simulink model "AssembledTEST1"  (R2016b)
settings: Solver=VariableStepAuto  StartTime=0.0  StopTime=60  RelTol=1e-9
values from neighbouring files (symbols this model uses):
  DOWN_0 = -xtrim(12)    [Comparison_NonLin.m]    (also in InitialiseJ31.m = 1830.0192; Trim.m)
  EAST_0 = xtrim(11)    [Comparison_NonLin.m]    (also in InitialiseJ31.m = 0; Trim.m)
  FLAP = 0    [InitialiseJ31.m]
  INERTIA = [IXX,IXY,IXZ;IXY,IYY,IYZ;IXZ,IYZ,IZZ]    [InitialiseJ31.m]
  NORTH_0 = xtrim(10)    [Comparison_NonLin.m]    (also in InitialiseJ31.m = 0; Trim.m)
  P_0 = xtrim(4)    [Comparison_NonLin.m]    (also in InitialiseJ31.m = 0; Trim.m)
  PHI_0 = xtrim(7)    [Comparison_NonLin.m]    (also in Trim.m)
  PSI_0 = xtrim(9)    [Comparison_NonLin.m]    (also in Trim.m)
  Q_0 = xtrim(5)    [Comparison_NonLin.m]    (also in InitialiseJ31.m = 0; Trim.m)
  R2D = 180/pi    (= 57.2957795131)    [InitialiseJ31.m]
  R_0 = xtrim(6)    [Comparison_NonLin.m]    (also in InitialiseJ31.m = 0; Trim.m)
  THETA_0 = xtrim(8)    [Comparison_NonLin.m]    (also in Trim.m)
  U_0 = xtrim(1)    [Comparison_NonLin.m]    (also in Trim.m)
  V_0 = xtrim(2)    [Comparison_NonLin.m]    (also in Trim.m)
  W_0 = xtrim(3)    [Comparison_NonLin.m]    (also in Trim.m)
undefined symbols (not defined in the file or in its folder): ail_data, Ap, Aw, b, beta0_data, c0, c_i, cdrag_data, CG, clean_wing_data, crt, CT_data, D, D0q_10, D0q_20, D0q_35, DCDi_data, DCM0b, Deh_f_on_data, Deh_on_data, df, Dqhq_data, e0, e_data10, e_data20, e_data35, elaw_0, elaw_1, elaw_2, flaps_lift_data, flaps_moment_data, flaps_tail_data, flaps_wing_data, fmc_data, fmf_data, fmn_data, fus_data, gamma_t, h_data10, h_data20, h_data35, it, iw, Iwn2, J_W, K1_data, k1f_data, k_data, L_r0_10f, L_r0_20f, L_r0_35f, l_t, ld_data, Lt, Lt_dash, Lv_b, Lv_h, Lv_n, mac, mach_ffr ... (+39)
libraries: aerolibasang x3, aerolibatmos2 x1
(part 5 of 5)

== matlab function AssembledTEST1/Subsystem/Lateral//Directional Aerodynamics/getYLN/Embedded MATLAB Function ==
  data: sigma input; Lv_b input; alpha input; Yv output; Yv_f input; Yv_v input; Y_rud input; Lv_di input; Lv_w_CL input; Np_w_CL input; Yp_w_CL input; a1_wb input; Lp_w input; CLw input; CLb input; Yv_wb input; Yv_n input; Yr_b input; Lv_n input; Lv_h input; Nv_wb input; Nv_n input; Nr_b input; J_W input; Yp output; Yr output; Y_zeta output; Lv output; Lp output; Lr output; L_zeta output; Nv output; Lr_0_f input; Lr_Lr0 input; Np output; Nr output; N_zeta output; b input; CD0w input; DelCDi_flap input; DelCD0_flap input
function [Yv,Yp,Yr,Y_zeta,Lv,Lp,Lr,L_zeta,Nv,Np,Nr,N_zeta] = Get_YLNderivs(sigma,Lv_b,alpha,Yv_f,Yv_v,Y_rud,Lv_di,Lv_w_CL,Np_w_CL,Yp_w_CL,a1_wb,Lp_w,CLw,CLb,Yv_wb,Yv_n,Yr_b,Lv_n,Lv_h,Nv_wb,Nv_n,Nr_b,J_W,Lr_0_f,Lr_Lr0,b,CD0w,DelCDi_flap,DelCD0_flap)

%CL_w,Dv_wing,D0_wing,p,q,r,Mach,V,alpha,beta,qbar,Aileron_L,Aileron_R,Rudder,Flap,wdot,xcg)

%   This function determines the side force, rolling momement and yawing
%   moment at the specified dynamic pressure.
%   Uses the methods given in ESDU 79006, 82010, 87008, 81013, 80033,
%   80034, 00025, 73006, A.06.01.03, 83006, 92029, 72021, 83026, 82017,
%   88029
%
%   Author: A Cooke Date:   1 Jun 05, modified 12 Jan 06, 16 Jun 06
%   Converted to embedded MatLab Function 31 Oct 07

% Yv_f  = sideforce derivative for fin 
Lv_f    =  (Yv_f/b) * (1.571 * cos(alpha) - 6.339 * sin(alpha));   % rolling moment derivative for fin
Nv_f    = -(Yv_f/b) * (6.339 * cos(alpha) + 1.571 * sin(alpha));   % yawing moment derivative for fin

% Yv_v  = sideforce derivative for ventral fin 
Lv_v    = -(Yv_v/b) * (0.524 * cos(alpha) + 6.335 * sin(alpha));   % rolling moment derivative for ventral fin 
Nv_v    = -(Yv_v/b) * (6.335 * cos(alpha) - 0.524 * sin(alpha));   % yawing moment derivative for ventral fin 

Yp_f    = -1.377 * (0.060 * cos(alpha) - 0.444 * sin(alpha) - 0.18 - sigma);  % sideforce derivative for fin
Lp_f    =  (Yp_f/b) * (0.946 * cos(alpha) - 7.042 * sin(alpha));     % rolling moment derivative for fin
Np_f    = -(Yp_f/b) * (7.042 * cos(alpha) + 0.946 * sin(alpha));     % yawing moment derivative for fin

Yr_f    = -(Yv_f/(b * J_W)) * (6.339 * cos(alpha) + 1.571 * sin(alpha));% sideforce derivative for fin
Lr_f    =  (Yr_f/b) * (1.571 * cos(alpha) - 6.339 * sin(alpha));        % rolling moment derivative for fin
Nr_f    = -(Yr_f/b) * (6.339 * cos(alpha) + 1.571 * sin(alpha));        % yawing moment derivative for fin

% Y_zeta  = sideforce derivative for rudder 
Y_zeta  = Y_rud * cos(32.3 * pi/180);      % conversion as rudder deflection normal to hinge line
L_zeta  =  (Y_zeta/b) * (1.498 * cos(alpha) - 6.833 * sin(alpha));  % rolling moment derivative for rudder
N_zeta  = -(Y_zeta/b) * (6.833 * cos(alpha) + 1.498 * sin(alpha));  % yawing moment derivative for rudder

DelCL_flap = CLw - CLb;   % determine increment in lift due to flap deployment        

Lv_w    = Lv_w_CL * CLb;                                 % rolling moment derivative from planform 
Yp_w    = Yp_w_CL * CLb;                                 % sideforce derivative from planform 
Np_w    = (Np_w_CL + 0.000038 * a1_wb) * CLb;            % yawing moment derivative from planform

Lv_flap = 0.0322 * DelCL_flap;                                 % rolling moment derivative from flap deployment 
Yv_flap = -DelCDi_flap + (0.045 * Yv_f + 0.003) * DelCL_flap;  % sideforce derivative from flap deployment
Nv_flap = 0.196 * DelCDi_flap + 0.045 * Nv_f * DelCL_flap;     % yawing moment derivative from flap deployment

Yp_di  =  0.3924 * Lp_w;                                % sideforce derivative from dihedral
Lp_di  = -0.0466 * Lp_w;                                % rolling moment derivative from dihedral
Np_di  =  0.0019 * Lp_w;                                % yawing moment derivative from dihedral

Nr_w = -0.1238 * (CD0w + 0.305 * DelCD0_flap) - 0.0053 * CLw^2; % yawing moment derivative from wing/flap

Lr_w    = (0.109 * CLw - 0.0037 + Lr_0_f) * Lr_Lr0;     % rolling moment derivative from wing/flap

% summation of derivatives

Yv      = Yv_wb + Yv_n + Yv_f + Yv_flap + Yv_v;
Yp      = Yp_w + Yp_di + Yp_f;
Yr      = Yr_b + Yr_f;

% Y_fin_w   = (qbar/V) * Sw * (Yv_f * v +  b * (Yp_f * p + Yr_f * r)) + Yrud * Rudder;    % total fin sideforce wind axes

Lv      = Lv_n + Lv_f + Lv_di + Lv_w + Lv_b + Lv_h + Lv_flap + Lv_v;
Lp      = Lp_w + Lp_di + Lp_f;
Lr      = Lr_w + Lr_f;

Nv      = Nv_wb + Nv_n + Nv_f + Nv_flap + Nv_v;
Np      = Np_w + Np_di + Np_f;
Nr      = Nr_w + Nr_b + Nr_f;

== matlab function AssembledTEST1/Subsystem/Lateral//Directional Aerodynamics/getYLN/Embedded MATLAB Function1 ==
  data: V input; alpha input; beta input; qbar input; Sw input; b input; Yv input; Y output; Yp input; Yr input; Yzeta input; Lv input; Lp input; Lr input; Lzeta input; Nv input; Np input; Nr input; Nzeta input; p input; r input; Rudder input; Nxi input; Lxi input; L output; N output
function [Y,L,N] = Get_YLN(V,alpha,beta,qbar,Sw,b,Yv,Yp,Yr,Yzeta,Lv,Lp,Lr,Lzeta,Nv,Np,Nr,Nzeta,p,r,Rudder,Nxi,Lxi)
% This function determines the lateral and driectional forces and moments

% written by A Cooke : 1 Nov 07

v       = V * sin(beta);

%---------- denormalising derivatives --------

Yv      = (qbar/V) * Sw * Yv;
Yp      = (qbar/V) * Sw * b * Yp;
Yr      = (qbar/V) * Sw * b * Yr;
Yzeta   = qbar * Sw * Yzeta;

Lv      = (qbar/V) * Sw * b * Lv;
Lp      = (qbar/V) * Sw * b^2 * Lp;
Lr      = (qbar/V) * Sw * b^2 * Lr;
Lrud    = qbar * Sw * b * Lzeta;
L_ail   = qbar * Sw * b * Lxi;                  % moment NOT derivative

Nv      = (qbar/V) * Sw * b * Nv;
Np      = (qbar/V) * Sw * b^2 * Np;
Nr      = (qbar/V) * Sw * b^2 * Nr;
Nrud    = qbar * Sw * b * Nzeta;
N_ail   = qbar * Sw * b * Nxi;                  % moment NOT derivative  


%---------- conversion to body axes ----------

Yv_by    = Yv;
Yrud_by  = Yzeta;
Yp_by    = Yp * cos(alpha) - Yr * sin(alpha);
Yr_by    = Yr * cos(alpha) + Yp * sin(alpha);

Y         = Yv_by * v + Yp_by * p + Yr_by * r + Yrud_by * Rudder; % total sideforce

Lv_by    = Lv * cos(alpha) - Nv * sin(alpha);
Lrud_by  = Lrud * cos(alpha) - Nrud * sin(alpha);
L_ail_by = L_ail * cos(alpha) - N_ail * sin(alpha);
Lp_by    = Lp * cos(alpha)^2 + Nr * sin(alpha)^2 - (Lr + Np) * sin(alpha) * cos(alpha);
Lr_by    = Lr * cos(alpha)^2 - Np * sin(alpha)^2 - (Lp - Nr) * sin(alpha) * cos(alpha);

Nv_by    = Nv * cos(alpha) + Lv * sin(alpha);
Nrud_by  = Nrud * cos(alpha) + Lrud * sin(alpha);
N_ail_by = N_ail * cos(alpha) + L_ail * sin(alpha);
Np_by    = Np * cos(alpha)^2 - Lr * sin(alpha)^2 + (Lp - Nr) * sin(alpha) * cos(alpha);
Nr_by    = Nr * cos(alpha)^2 + Lp * sin(alpha)^2 + (Lr + Np) * sin(alpha) * cos(alpha);

L       = Lv_by * v + Lr_by * r + Lp_by * p + Lrud_by * Rudder + L_ail_by; % total rolling moment
N       = Nv_by * v + Nr_by * r + Np_by * p + Nrud_by * Rudder + N_ail_by; % total yawing moment

== matlab function AssembledTEST1/Subsystem/Longitudinal Aerodynamics/Get Drag/Embedded MATLAB Function ==
  data: Sw input; qh_q output; Aw input; mac input; Lt input; gamma_t input; alpha_w input; Dqw input; CLw input
function qh_q = Get_qhq(Sw,Aw,mac,Lt,gamma_t,alpha_w,Dqw,CLw)

% this function determines the power-off dynamic pressure at
% the tailplane using NASA TN D-6800

% written by A Cooke - 12 Sep 07

CDw = Dqw/Sw;
eh  = (1.62 * CLw)/(pi * Aw);   % downwash in plane of symmetry
mu  = gamma_t + eh - alpha_w;

X = Lt * cos(mu);
Z = Lt * sin(mu);

delZ_mac = 0.68 * sqrt(CDw * ((X/mac) + 0.15));
delZ     = delZ_mac * mac;

delq_q0  = (2.42 * sqrt(CDw))/((X/mac) + 0.3);

if (Z/delZ) > 1.0
    delq_q = 0.0;
else
    delq_q = delq_q0 * (cos((pi/2)*(Z/delZ)))^2;
end

qh_q = 1 - delq_q;

== matlab function AssembledTEST1/Subsystem/Powerplants and Slipstream/Subsystem2/Powerplant - port (forces and moments about spinner) (in body axes)/Embedded MATLAB Function ==
  data: Xp_dash input; Ai output; Zt_dash input; Dp input; c_i input; alpha_b input; upwash input; downwash_p input; Si output
function [Ai,Si] = GetARimmersed(Xp_dash,Zt_dash,Dp,c_i,alpha_b,upwash,downwash_p)

% This fuction detemines the aspect ratio of the portion of the wing
% immersed in the propeller slipstream. Taken from NASA TN D-6800

% written by A Cooke 3 Aug 07

Zs_dash = Zt_dash + Xp_dash * tan(alpha_b + upwash - downwash_p);
b_i     = 2 * sqrt((Dp/2)^2 + Zs_dash^2);
Ai      = b_i/c_i;
Si      = b_i*c_i;

== matlab function AssembledTEST1/Subsystem/Powerplants and Slipstream/Subsystem2/Powerplant - port (forces and moments about spinner) (in body axes)/Embedded MATLAB Function1 ==
  data: deuda input; CLw input; Sw input; TC input; K1 input; Si input; ep input; DCLw_slip output; D0qw_slip output; D0qw input; a1 input
function [DCLw_slip,D0qw_slip] = Get_CLD0qw_slip(deuda,CLw,Sw,TC,K1,Si,ep,D0qw,a1)

% Thus function determines the contribution to wing CL and D0/q made by
% the propeller slipstream using NASA TN D-6800

% written by A Cooke: 14 Aug 07, modified 24 Jan 08

delqbarw_qbar = TC * 8/pi;
delalpha_si   = -ep/(1 - deuda);

D0qw_slip = D0qw * (Si/Sw) * delqbarw_qbar;
DCLw_slip = CLw * (Si/Sw) * K1 * delqbarw_qbar;
DCLw_slip = DCLw_slip + ((Si/Sw) * a1 * delalpha_si * (1 + delqbarw_qbar));

== matlab function AssembledTEST1/Subsystem/Powerplants and Slipstream/Subsystem2/Embedded MATLAB Function ==
  data: X input; L output; Y input; Z input; xyz input; M output; N output
function [L,M,N] = getLMN(X,Y,Z,xyz)
% This block converts propeller forces into moments
% about the Body Axes Centre

x = xyz(1);
y = xyz(2);
z = xyz(3);
L = Z*y - Y*z;
M = X*z - Z*x;
N = Y*x - X*y;

== matlab function AssembledTEST1/Subsystem/Powerplants and Slipstream/Subsystem2/Embedded MATLAB Function1 ==
  data: X input; L output; Y input; Z input; xyz input; M output; N output
function [L,M,N] = getLMN(X,Y,Z,xyz)
% This block converts propeller forces into moments
% about the Body Axes Centre

x = xyz(1);
y = xyz(2);
z = xyz(3);
L = Z*y - Y*z;
M = X*z - Z*x;
N = Y*x - X*y;

== matlab function AssembledTEST1/Subsystem/Powerplants and Slipstream/Subsystem2/Embedded MATLAB Function2 ==
  data: Cm0w input; Cm0i output; Sw input; mac input; b input; S_ip input; S_is input; c_i input
function Cm0i = getCm0i(Cm0w,Sw,mac,b,S_ip,S_is,c_i)

% This function determines the zero lift pitching moment of the 
% basic wing for that portion not influenced by the propeller slipstreams

% written by A Cooke : 9 Oct 07

b_ip = S_ip/c_i;
b_is = S_is/c_i;

Cm0i = Cm0w*(1 - (((Sw - S_ip - S_is)^2)/(Sw*mac*(b - b_ip - b_is))));

== matlab function AssembledTEST1/Subsystem/Powerplants and Slipstream/Subsystem2/Embedded MATLAB Function3 ==
  data: X output; Lift input; Drag input; Pitch input; alpha input; Y output; Z output; L output; M output; N output; x input; z input; xyz input
function [X,Y,Z,L,M,N]  = getSlipFM(Lift,Drag,Pitch,alpha,x,z,xyz)
% This function converts the increments in lift, drag
% and pitching moment for the wing caused by the 
% propellor slipstream into forces and moments at 
% the body axes centre

% written by A Cooke : 16 Oct 07

x = xyz(1) - x;
y = xyz(2);
z = xyz(3) + z;
X =  Lift * sin(alpha) - Drag * cos(alpha);
Y = 0.0;
Z = -Lift * cos(alpha) - Drag * sin(alpha);
L = Z*y - Y*z;
M = X*z - Z*x + Pitch;
N = Y*x - X*y;

== matlab function AssembledTEST1/Subsystem/Powerplants and Slipstream/Subsystem2/Embedded MATLAB Function4 ==
  data: X output; Lift input; Drag input; Pitch input; alpha input; Y output; Z output; L output; M output; N output; x input; z input; xyz input
function [X,Y,Z,L,M,N]  = getSlipFM(Lift,Drag,Pitch,alpha,x,z,xyz)
% This function converts the increments in lift, drag
% and pitching moment for the wing caused by the 
% propellor slipstream into forces and moments at 
% the body axes centre

% written by A Cooke : 16 Oct 07

x = xyz(1) - x;
y = xyz(2);
z = xyz(3) + z;
X =  Lift * sin(alpha) - Drag * cos(alpha);
Y = 0.0;
Z = -Lift * cos(alpha) - Drag * sin(alpha);
L = Z*y - Y*z;
M = X*z - Z*x + Pitch;
N = Y*x - X*y;

== matlab function AssembledTEST1/Subsystem/Powerplants and Slipstream/Subsystem2/Get_delDi/GetDelCDi ==
  data: KDi input; alpha input; delDi output; bar_e_ep input; Xp input; Zp input; CLw input; deu_dap input; qbar input; Sw input; Aw input; b input; CDiw input; D input
function delDi = getDelDi(KDi,alpha,bar_e_ep,Xp,Zp,CLw,deu_dap,qbar,Sw,Aw,b,CDiw,D)
% This block estimates DelCDi using method from NASA TN D-6800
% written by: A Cooke -  22 Oct 07

CL_ddash = CLw + ((Xp * sin(alpha) - Zp * cos(alpha))/(qbar * Sw));
ebar     = bar_e_ep * deu_dap * alpha;
factor1  = ((CLw/CL_ddash)^2)*(1 + (pi* Aw *ebar)/CLw);
factor2  = ((b/D) * ((Xp * sin(alpha) - Zp * cos(alpha))/(qbar * Sw * CL_ddash)))^2;
delCDi   = CDiw * (factor1 + (KDi * factor2) - 1);
delDi    = delCDi * Sw * qbar;

== matlab function AssembledTEST1/Subsystem/Powerplants and Slipstream/Subsystem2/Get_delDi1/GetDelCDi ==
  data: KDi input; alpha input; delDi output; bar_e_ep input; Xp input; Zp input; CLw input; deu_dap input; qbar input; Sw input; Aw input; b input; CDiw input; D input
function delDi = getDelDi(KDi,alpha,bar_e_ep,Xp,Zp,CLw,deu_dap,qbar,Sw,Aw,b,CDiw,D)
% This block estimates DelCDi using method from NASA TN D-6800
% written by: A Cooke -  22 Oct 07

CL_ddash = CLw + ((Xp * sin(alpha) - Zp * cos(alpha))/(qbar * Sw));
ebar     = bar_e_ep * deu_dap * alpha;
factor1  = ((CLw/CL_ddash)^2)*(1 + (pi* Aw *ebar)/CLw);
factor2  = ((b/D) * ((Xp * sin(alpha) - Zp * cos(alpha))/(qbar * Sw * CL_ddash)))^2;
delCDi   = CDiw * (factor1 + (KDi * factor2) - 1);
delDi    = delCDi * Sw * qbar;

== matlab function AssembledTEST1/Subsystem/Powerplants and Slipstream/Subsystem2/Embedded MATLAB Function5 ==
  data: Cm0i input; Sw input; S_i input; mac input; c_i input; DelCM output; TC input; DelCL input; xw input
function DelCM = getDelCm(Cm0i,Sw,S_i,mac,c_i,TC,DelCL,xw)

% This function determines the pitching moment increment 
% caused by the propeller slipstream

% written by A Cooke : 23 Oct 07

Del_qw_qbar = TC * 8/pi;

DelCM0_qw = Del_qw_qbar * (S_i/Sw) * (c_i/mac) * Cm0i;
DelCM_wL  = -DelCL * (xw/mac);
DelCM = DelCM0_qw + DelCM_wL;

== matlab function AssembledTEST1/Subsystem/Powerplants and Slipstream/Subsystem2/Powerplant - port (forces and moments about spinner) (in body axes)/Get_Del_qhq/Embedded MATLAB Function ==
  data: Flap input; Del_eh_power output; Deh_power input; Deh_power_flap input
function Del_eh_power = Get_Del_eh(Flap,Deh_power,Deh_power_flap)

if Flap > 0
   Del_eh_power = Deh_power_flap;
else
   Del_eh_power = Deh_power;
end

== matlab function AssembledTEST1/Subsystem/Powerplants and Slipstream/Subsystem2/Powerplant - port (forces and moments about spinner) (in body axes)/Get_Del_qhq/Embedded MATLAB Function1 ==
  data: ep input; DelMp_q output; eu input; TC input; Iwn2 input
function DelMp_q = getDelMp(ep,eu,TC,Iwn2)
% This block determines the change in free moments for the
% nacelle due to slipstream effects, see NASA TN D-6800

% Author: A Cooke - 26 Oct 07

Del_qw_q = TC * 8/pi;
DelMp_q = (180/pi)*(eu - ep)*(1 + Del_qw_q)*Iwn2/36.5;

== matlab function AssembledTEST1/Subsystem/Powerplants and Slipstream/Subsystem2/Embedded MATLAB Function6 ==
  data: Cm0i input; Sw input; S_i input; mac input; c_i input; DelCM output; TC input; DelCL input; xw input
function DelCM = getDelCm(Cm0i,Sw,S_i,mac,c_i,TC,DelCL,xw)

% This function determines the pitching moment increment 
% caused by the propeller slipstream

% written by A Cooke : 23 Oct 07

Del_qw_qbar = TC * 8/pi;

DelCM0_qw = Del_qw_qbar * (S_i/Sw) * (c_i/mac) * Cm0i;
DelCM_wL  = -DelCL * (xw/mac);
DelCM = DelCM0_qw + DelCM_wL;

== matlab function AssembledTEST1/Subsystem/Powerplants and Slipstream/Subsystem2/Embedded MATLAB Function7 ==
  data: Lift input; X output; Drag input; alpha input; x input; y input; z input; Y output; Z output; L output; M output; N output
function [X,Y,Z,L,M,N]  = getSlipFMt(Lift,Drag,alpha,x,y,z)
% This function converts the increments in lift, drag
% and pitching moment for the tail caused by the 
% propellor slipstream into forces and moments at 
% the body axes centre

% written by A Cooke : 22 Nov 07

X =  Lift * sin(alpha) - Drag * cos(alpha);
Y = 0.0;
Z = -Lift * cos(alpha) - Drag * sin(alpha);
L = Z*y - Y*z;
M = X*z - Z*x;
N = Y*x - X*y;

== matlab function AssembledTEST1/Subsystem/Powerplants and Slipstream/Subsystem2/Embedded MATLAB Function8 ==
  data: Lift input; X output; Drag input; alpha input; x input; y input; z input; Y output; Z output; L output; M output; N output
function [X,Y,Z,L,M,N]  = getSlipFMt(Lift,Drag,alpha,x,y,z)
% This function converts the increments in lift, drag
% and pitching moment for the tail caused by the 
% propellor slipstream into forces and moments at 
% the body axes centre

% written by A Cooke : 22 Nov 07

X =  Lift * sin(alpha) - Drag * cos(alpha);
Y = 0.0;
Z = -Lift * cos(alpha) - Drag * sin(alpha);
L = Z*y - Y*z;
M = X*z - Z*x;
N = Y*x - X*y;

== matlab function AssembledTEST1/Subsystem/Powerplants and Slipstream/Subsystem2/Powerplant - port (forces and moments about spinner) (in body axes)/Propeller - left (forces and moments about spinner) (in body axes)/Embedded MATLAB Function ==
  data: CT input; beta0 input; sigma_e input; CZ_alpha output; CN_alpha output; J input
function [CZ_alpha,CN_alpha] = PropDevs(CT,beta0,sigma_e,J)

% This function determines the propeller derivatives
% at the specified Power Coefficient and Advance Ratio
%
% Author: A Cooke Date: 7 Jun 06, modified 26 Oct 06

Tc = CT * 8/(pi * J^2);
kb = tan(d2r(beta0 - 5))/(sigma_e * cos(d2r(beta0 - 5)));
CZ_alpha = -((4.25 * sigma_e)/(1 + 2 * sigma_e)) * sin(d2r(beta0 + 3)) * (1 + ((3 * Tc/8)/sqrt(1 + (2*Tc/3))));
CZ_alpha = CZ_alpha * (CT/Tc);
CN_CZ    = -(0.321/(sigma_e + tan(d2r(beta0 + 5)))) * (1 + ((Tc * kb/3)/(1 + (3 * Tc * sqrt(kb)/4))));
CN_alpha = CN_CZ * CZ_alpha;

function rad = d2r(deg)

%   This function converts degrees to radians
%
%   Author: A Cooke Date: 5 May 2004

rad = deg * pi/180;

== matlab function AssembledTEST1/Subsystem/Powerplants and Slipstream/Subsystem2/Powerplant - starboard (forces and moments about spinner) (in body axes)/Embedded MATLAB Function ==
  data: Xp_dash input; Ai output; Zt_dash input; Dp input; c_i input; alpha_b input; upwash input; downwash_p input; Si output
function [Ai,Si] = GetARimmersed(Xp_dash,Zt_dash,Dp,c_i,alpha_b,upwash,downwash_p)

% This fuction detemines the aspect ratio of the portion of the wing
% immersed in the propeller slipstream. Taken from NASA TN D-6800

% written by A Cooke 3 Aug 07

Zs_dash = Zt_dash + Xp_dash * tan(alpha_b + upwash - downwash_p);
b_i     = 2 * sqrt((Dp/2)^2 + Zs_dash^2);
Ai      = b_i/c_i;
Si      = b_i*c_i;

== matlab function AssembledTEST1/Subsystem/Powerplants and Slipstream/Subsystem2/Powerplant - starboard (forces and moments about spinner) (in body axes)/Embedded MATLAB Function1 ==
  data: deuda input; CLw input; Sw input; TC input; K1 input; Si input; ep input; DCLw_slip output; D0qw_slip output; D0qw input; a1 input
function [DCLw_slip,D0qw_slip] = Get_CLD0qw_slip(deuda,CLw,Sw,TC,K1,Si,ep,D0qw,a1)

% Thus function determines the contribution to wing CL and D0/q made by
% the propeller slipstream using NASA TN D-6800

% written by A Cooke: 14 Aug 07, modified 24 Jan 08

delqbarw_qbar = TC * 8/pi;
delalpha_si   = -ep/(1 - deuda);

D0qw_slip = D0qw * (Si/Sw) * delqbarw_qbar;
DCLw_slip = CLw * (Si/Sw) * K1 * delqbarw_qbar;
DCLw_slip = DCLw_slip + ((Si/Sw) * a1 * delalpha_si * (1 + delqbarw_qbar));

== matlab function AssembledTEST1/Subsystem/Powerplants and Slipstream/Subsystem2/Powerplant - starboard (forces and moments about spinner) (in body axes)/Get_Del_qhq/Embedded MATLAB Function ==
  data: Flap input; Del_eh_power output; Deh_power input; Deh_power_flap input
function Del_eh_power = Get_Del_eh(Flap,Deh_power,Deh_power_flap)

if Flap > 0
   Del_eh_power = Deh_power_flap;
else
   Del_eh_power = Deh_power;
end

== matlab function AssembledTEST1/Subsystem/Lateral//Directional Aerodynamics/getYLN/get_n_xi/Embedded MATLAB Function ==
  data: xi_s input; C_np output; xi_p input
function C_np = get_Cnp(xi_s,xi_p)
% This block outputs the yaw moment coefficient due to the profile drag casued by
% aileron deflection, uses ESDU 88029

% written by A Cooke: 10 Jan 08

if xi_s == 0.0
    if xi_p == 0.0
        C_np = 0.0;
    else
        C_np = 0.0119 * (0.0 - (1 - 0.0665 * (1 + (abs(xi_p)/xi_p)))*(0.0897 - xi_p)^2);
    end
elseif xi_p == 0.0
    C_np    = 0.0119 * ((1 - 0.0665 * (1 - (abs(xi_s)/xi_s)))*(0.0897 + xi_s)^2 - 0.0);
else
C_np    = 0.0119 * ((1 - 0.0665 * (1 - (abs(xi_s)/xi_s)))*(0.0897 + xi_s)^2 - (1 - 0.0665 * (1 + (abs(xi_p)/xi_p)))*(0.0897 - xi_p)^2);
end

== matlab function AssembledTEST1/Subsystem/Longitudinal Aerodynamics/Get Fuselage XZM/Embedded MATLAB Function ==
  data: Dq input; Mq input; CN input; CM input; X output; qbar input; q input; Sref input; df input; Sw input; mac input; CM0 input; Z output; M output
function [X,Z,M] = Get_XZMfus(Dq,Mq,CN,CM,qbar,q,Sref,df,Sw,mac,CM0)

% This function determines the fuselage contribution to the
% X force, Z force and M moment.

% written by A Cooke, 16 Jan 10

X  = -qbar * Dq;
Z  = -qbar * Sref * CN;
M  = -qbar * Sref * CM * df;
M0 = mac * qbar * Sw * CM0;
M  = M + M0 + (Mq * q * qbar * Sw * mac^2);

return

== matlab function AssembledTEST1/Subsystem/Lateral//Directional Aerodynamics/getYLN/slipstream effects ==
  data: b input; Xp_dash input; xp input; yp input; Xp input; Yv_ns output; Lv_s output; Lp_s output; Lr_s output; deu_dap input; DCLw input; Yv_n input; Nv_n input; qbar input; D input; Nv_ns output
function [Yv_ns,Lv_s,Lp_s,Lr_s,Nv_ns] = Get_YLNslip(b,Xp_dash,xp,yp,Xp,deu_dap,DCLw,Yv_n,Nv_n,qbar,D)
% This block estimates the slipstream effect on lateral and directional
% aeroderivatves using NASA TN D-6946

% written by A Cooke 24 Jan 08

Del_qbar_ratio = (4 * Xp)/(qbar * pi * D^2);
slip_factor    = Del_qbar_ratio - deu_dap*(1 + Del_qbar_ratio);

Yv_ns = Yv_n * slip_factor;
Nv_ns = Nv_n * slip_factor;
Lv_s  = 0.5 * (Xp_dash/b) * DCLw * (1 - deu_dap);
Lp_s  = -4 * DCLw * (yp/b)^2;
Lr_s  =  2 * DCLw * (xp/b)^2;

== matlab function AssembledTEST1/Subsystem/Powerplants and Slipstream/Subsystem2/Powerplant - starboard (forces and moments about spinner) (in body axes)/Get_Del_qhq/Embedded MATLAB Function1 ==
  data: ep input; DelMp_q output; eu input; TC input; Iwn2 input
function DelMp_q = getDelMp(ep,eu,TC,Iwn2)
% This block determines the change in free moments for the
% nacelle due to slipstream effects, see NASA TN D-6800

% Author: A Cooke - 26 Oct 07

Del_qw_q = TC * 8/pi;
DelMp_q = (180/pi)*(eu - ep)*(1 + Del_qw_q)*Iwn2/36.5;

== matlab function AssembledTEST1/Subsystem/Powerplants and Slipstream/Subsystem2/Powerplant - starboard (forces and moments about spinner) (in body axes)/Propeller - right (forces and moments about spinner) (in body axes)/Embedded MATLAB Function ==
  data: CT input; beta0 input; sigma_e input; CZ_alpha output; CN_alpha output; J input
function [CZ_alpha,CN_alpha] = PropDevs(CT,beta0,sigma_e,J)

% This function determines the propeller derivatives
% at the specified Power Coefficient and Advance Ratio
%
% Author: A Cooke Date: 7 Jun 06, modified 26 Oct 06

Tc = CT * 8/(pi * J^2);
kb = tan(d2r(beta0 - 5))/(sigma_e * cos(d2r(beta0 - 5)));
CZ_alpha = -((4.25 * sigma_e)/(1 + 2 * sigma_e)) * sin(d2r(beta0 + 3)) * (1 + ((3 * Tc/8)/sqrt(1 + (2*Tc/3))));
CZ_alpha = CZ_alpha * (CT/Tc);
CN_CZ    = -(0.321/(sigma_e + tan(d2r(beta0 + 5)))) * (1 + ((Tc * kb/3)/(1 + (3 * Tc * sqrt(kb)/4))));
CN_alpha = CN_CZ * CZ_alpha;

function rad = d2r(deg)

%   This function converts degrees to radians
%
%   Author: A Cooke Date: 5 May 2004

rad = deg * pi/180;

== matlab function AssembledTEST1/Equations of Motion/Rotational_Kinematic_Transform ==
  data: angles input; rates input; anglesDot output
function anglesDot   = rotationalkinematic(angles, rates)

phi = angles(1);
theta = angles(2);

P = rates(1);
Q = rates(2);
R = rates(3);

transfMat = [1, sin(phi).*tan(theta), cos(phi).*tan(theta);...
			0, cos(phi), -sin(phi);...
			0, sin(phi).*sec(theta), cos(phi).*sec(theta)];

anglesDot = transfMat*[P; Q; R];

end

== matlab function AssembledTEST1/Gravitational_Forces_Moments ==
  data: angles input; d input; mass input; Fg output; Mg output
function [Fg, Mg] = gravityFn(angles, d, mass)

dx = d(1);
dy = d(2);
dz = d(3);

phi = angles(1);
theta = angles(2);

gMat = [-mass*9.81*sin(theta);
		mass*9.81*sin(phi)*cos(theta);
		mass*9.81*cos(phi)*cos(theta)];

mat = [1, 0, 0;
		0, 1, 0;
		0, 0, 1;
		0, -dz, dy;
		dz, 0, -dx; % it is wrong in the notes, there, the terms are swapped and dx does not have the "minus sign"
		-dy, dx, 0];
    
X = mat*gMat;

Fg = [X(1); X(2); X(3)];
Mg = [X(4); X(5); X(6)];
end
